simulink model "SMOModel"  (R2021a)
settings: Solver=VariableStepAuto  StartTime=0.0  StopTime=6  RelTol=1e-3
settings Model: Creator=abang  LastModifiedBy=abang

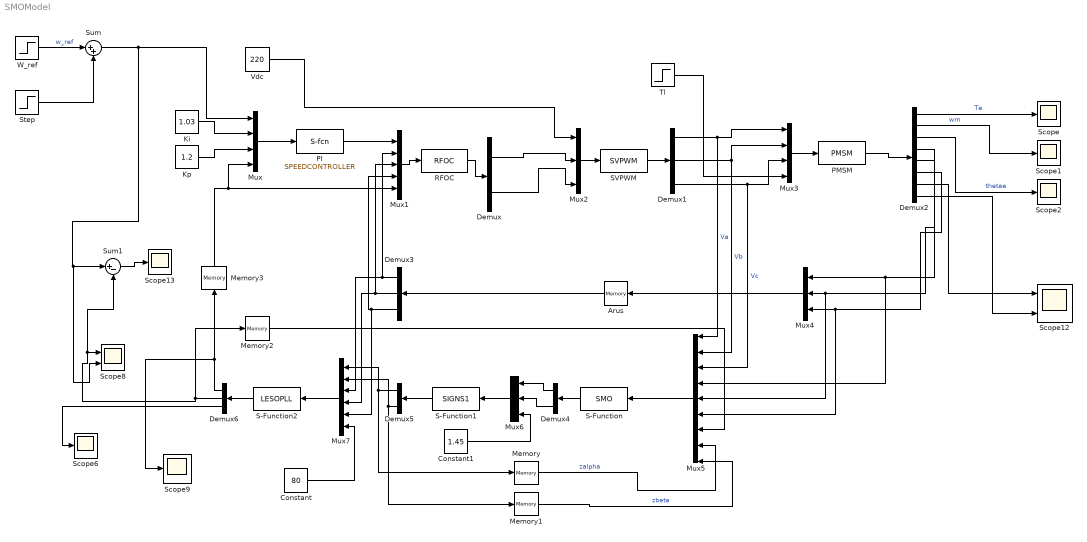
== system SMOModel ==
  Arus : Memory
  Constant : Constant  Value=80
  Constant1 : Constant  Value=1.45
  Demux : Demux  Outputs=2
  Demux1 : Demux  Outputs=3
  Demux2 : Demux  Outputs=8
  Demux3 : Demux  Outputs=3
  Demux4 : Demux  Outputs=2
  Demux5 : Demux  Outputs=2
  Demux6 : Demux  Outputs=3
  Ki : Constant  Value=1.03
  Kp : Constant  Value=1.2
  Memory{,1..3} (4 alike) : Memory
  Mux : Mux
  Mux1 : Mux  Inputs=5
  Mux2 : Mux  Inputs=3
  Mux3 : Mux
  Mux4 : Mux  Inputs=3
  Mux5 : Mux  Inputs=9
  Mux6 : Mux  Inputs=3
  Mux7 : Mux  Inputs=6
  PI : S-Function  FunctionName=SPEEDCONTROLLER  SFunctionDeploymentMode=off  EnableBusSupport=off
  PMSM : S-Function  FunctionName=PMSM  SFunctionDeploymentMode=off  EnableBusSupport=off
  RFOC : S-Function  FunctionName=RFOC  SFunctionDeploymentMode=off  EnableBusSupport=off
  S-Function : S-Function  FunctionName=SMO  SFunctionDeploymentMode=off  EnableBusSupport=off
  S-Function1 : S-Function  FunctionName=SIGNS1  SFunctionDeploymentMode=off  EnableBusSupport=off
  S-Function2 : S-Function  FunctionName=LESOPLL  SFunctionDeploymentMode=off  EnableBusSupport=off
  SVPWM : S-Function  FunctionName=SVPWM  SFunctionDeploymentMode=off  EnableBusSupport=off
  Scope{,1..2,6,9,13} (6 alike) : Scope
  Scope12 : Scope  NumInputPorts=2
  Scope8 : Scope  NumInputPorts=2
  Step : Step  Time=4  After=30  SampleTime=0
  Sum : Sum  Inputs=|++
  Sum1 : Sum  Inputs=|+-
  Tl : Step  Time=9  After=0  SampleTime=0
  Vdc : Constant  Value=220
  W_ref : Step  Time=2  Before=30  After=60  SampleTime=0.00001
  wires:
  Mux/1 -> PI/1
  Mux2/1 -> SVPWM/1
  SVPWM/1 -> Demux1/1
  Mux3/1 -> PMSM/1
  Ki/1 -> Mux/2
  Kp/1 -> Mux/3
  RFOC/1 -> Demux/1
  Mux1/1 -> RFOC/1
  PI/1 -> Mux1/1
  Vdc/1 -> Mux2/1
  Demux3/1 -> Mux7/3, Mux1/2
  Demux3/2 -> Mux7/4, Mux1/3
  Demux3/3 -> Mux7/5, Mux1/4
  Mux4/1 -> Arus/1
  Arus/1 -> Demux3/1
  Demux/1 -> Mux2/2
  Mux5/1 -> S-Function/1
  S-Function/1 -> Demux4/1
  Demux4/1 -> Mux6/1
  Demux4/2 -> Mux6/2
  Mux6/1 -> S-Function1/1
  S-Function1/1 -> Demux5/1
  Demux5/1 -> Memory/1, Mux7/1
  Memory/1 -> Mux5/8  "zalpha"
  Demux5/2 -> Mux7/2, Memory1/1
  Memory1/1 -> Mux5/9  "zbeta"
  Mux7/1 -> S-Function2/1
  S-Function2/1 -> Demux6/1
  Demux6/1 -> Scope9/1, Memory3/1
  Memory3/1 -> Mux/4, Mux1/5
  Constant/1 -> Mux7/6
  Demux/2 -> Mux2/3
  Constant1/1 -> Mux6/3
  Demux1/1 -> Mux3/1, Mux5/1  "Va"
  Demux1/2 -> Mux3/2, Mux5/2  "Vb"
  Demux1/3 -> Mux5/3, Mux3/3  "Vc"
  Tl/1 -> Mux3/4
  PMSM/1 -> Demux2/1
  Demux2/1 -> Scope/1  "Te"
  Demux2/2 -> Scope1/1  "wm"
  Demux2/3 -> Scope2/1  "thetae"
  Demux2/4 -> Mux5/4, Mux4/1
  Demux2/5 -> Mux5/5, Mux4/2
  Demux2/6 -> Mux5/6, Mux4/3
  W_ref/1 -> Sum/1  "w_ref"
  Demux6/3 -> Scope6/1
  Memory2/1 -> Mux5/7
  Demux2/7 -> Scope12/1
  Demux2/8 -> Scope12/2
  Sum1/1 -> Scope13/1
  Demux6/2 -> Scope8/1, Sum1/2, Memory2/1
  Sum/1 -> Scope8/2, Sum1/1, Mux/1
  Step/1 -> Sum/2
